simulink model "sl_bicycle"  (Simulink 7.6)
settings: Solver=ode45  StartTime=0.0  StopTime=10.0  RelTol=1e-3
libraries: roblocks x1
settings Model: Creator=pic  LastModifiedBy=n6334687
settings DebuggingCC: StrictBusMsg=Warning

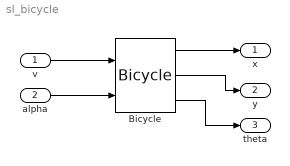
== system sl_bicycle ==
  v : Inport
  alpha : Inport  Port=2
  Bicycle : roblocks/Dynamics/Bicycle  SystemSampleTime=-1  accel=1  vlim=1  alim=2  x0=[0, 0, 0]  handbrake=0
  x : Outport
  y : Outport  Port=2
  theta : Outport  Port=3
  wires:
  v/1 -> Bicycle/1
  alpha/1 -> Bicycle/2
  Bicycle/1 -> x/1
  Bicycle/2 -> y/1
  Bicycle/3 -> theta/1
